simulink model "moteur"  (R2018a)
settings: Solver=VariableStepAuto  StartTime=0.0  StopTime=10.0  RelTol=1e-3
values from neighbouring files (symbols this model uses):
  Cr = 0.02068    [moteur_bf.m]    (also in moteur_bf2.m)
  E = 50    [moteur_bf.m]    (also in moteur_bf2.m)
  f = 6.79e-5    (= 6.79e-05)    [moteur_bf.m]    (also in moteur_bf2.m)
  J = 1.37e-4    (= 0.000137)    [moteur_bf.m]    (also in moteur_bf2.m)
  k = 0.209    [moteur_bf.m]    (also in moteur_bf2.m)
  Kc = 5.5    [moteur_bf.m]    (also in moteur_bf2.m)
  Kd = 1    [moteur_bf2.m]
  Ki = 0    [moteur_bf.m]    (also in moteur_bf2.m = 2)
  Kp = 1    [moteur_bf.m]    (also in moteur_bf2.m = 4)
  L = 1e-3    (= 0.001)    [moteur_bf.m]    (also in moteur_bf2.m)
  R = 5    [moteur_bf.m]    (also in moteur_bf2.m)
libraries: simulink x1
settings Model: Creator=tomto  LastModifiedBy=Thomas

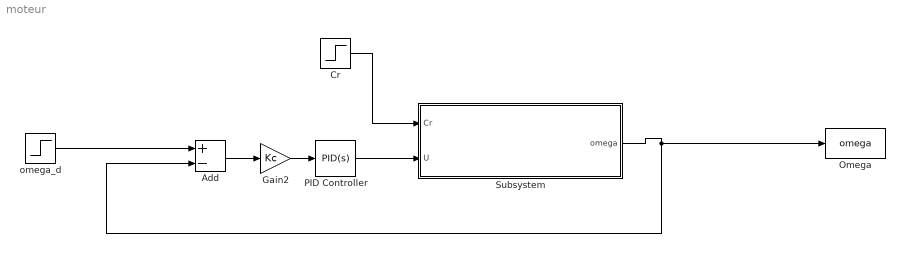
== system moteur ==
  Add : Sum  Inputs=+-
  Cr : Step  Time=2.5  After=Cr  SampleTime=0
  Gain2 : Gain  Gain=Kc
  Omega : ToWorkspace  VariableName=omega  SaveFormat=Timeseries  SampleTime=-1
  PID Controller : simulink/Continuous/PID Controller  Controller=PID  TimeDomain=Continuous-time  SampleTime=-1  IntegratorMethod=Forward Euler  FilterMethod=Forward Euler  Form=Parallel  UseFilter=off  ControllerParametersSource=internal  P=Kp  I=Ki  D=Kd  N=1  InitialConditionSource=internal  InitialConditionForIntegrator=Ki  InitialConditionForFilter=1  ExternalReset=none  LimitOutput=off  UpperSaturationLimit=inf  LowerSaturationLimit=-inf  LinearizeAsGain=on  AntiWindupMode=none  Kb=1  TrackingMode=off  Kt=1  PParamMin=[]  PParamMax=[]  IParamMin=[]  IParamMax=[]  DParamMin=[]  DParamMax=[]  NParamMin=[]  NParamMax=[]  KbParamMin=[]  KbParamMax=[]  KtParamMin=[]  KtParamMax=[]  POutMin=[]  POutMax=[]  IOutMin=[]  IOutMax=[]  DOutMin=[]  DOutMax=[]  NOutMin=[]  NOutMax=[]  KbOutMin=[]  KbOutMax=[]  KtOutMin=[]  KtOutMax=[]  IntegratorOutMin=[]  IntegratorOutMax=[]  FilterOutMin=[]  FilterOutMax=[]  SumOutMin=[]  SumOutMax=[]  SumI1OutMin=[]  SumI1OutMax=[]  SumI2OutMin=[]  SumI2OutMax=[]  SumI3OutMin=[]  SumI3OutMax=[]  SumDOutMin=[]  SumDOutMax=[]  SaturationOutMin=[]  SaturationOutMax=[]  IntegratorContinuousStateAttributes=''  IntegratorStateMustResolveToSignalObject=off  IntegratorRTWStateStorageClass=Auto  FilterContinuousStateAttributes=''  FilterStateMustResolveToSignalObject=off  FilterRTWStateStorageClass=Auto  DifferentiatorICPrevScaledInput=0  DifferentiatorOutMin=[]  DifferentiatorOutMax=[]  FilterDiffOutCoefMin=[]  FilterDiffOutCoefMax=[]  SumDenOutMin=[]  SumDenOutMax=[]  SumNumOutMin=[]  SumNumOutMax=[]  ReciprocalOutMin=[]  ReciprocalOutMax=[]  DivideOutMin=[]  DivideOutMax=[]  TunerSelectOption=Transfer Function Based (PID Tuner App)
  Subsystem : Subsystem
  omega_d : Step  Time=0  After=E  SampleTime=0
  wires:
  Cr/1 -> Subsystem/1(Cr)
  omega_d/1 -> Add/1
  Subsystem/1(omega) -> Add/2, Omega/1
  PID Controller/1 -> Subsystem/2(U)
  Add/1 -> Gain2/1
  Gain2/1 -> PID Controller/1

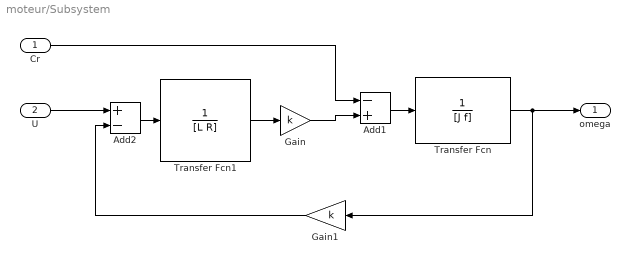
== system moteur/Subsystem ==
  Cr : Inport
  U : Inport  Port=2
  Add1 : Sum  Inputs=-+
  Add2 : Sum  Inputs=+-
  Gain : Gain  Gain=k
  Gain1 : Gain  Gain=k
  Transfer Fcn : TransferFcn  Denominator=[J f]
  Transfer Fcn1 : TransferFcn  Denominator=[L R]
  omega : Outport
  wires:
  Gain1/1 -> Add2/2
  Gain/1 -> Add1/2
  Add2/1 -> Transfer Fcn1/1
  Add1/1 -> Transfer Fcn/1
  Transfer Fcn/1 -> omega/1, Gain1/1
  Transfer Fcn1/1 -> Gain/1
  Cr/1 -> Add1/1
  U/1 -> Add2/1
